simulink model "brain"  (Simulink 7.5)
settings: Solver=FixedStepDiscrete  StartTime=0.0  StopTime=inf  FixedStep=0.2  RelTol=1e-3
values from neighbouring files (symbols this model uses):
  Buoy1_Hue = 0.4    [brainconstants.m]    (also in brainconstants_David.m = 30)
  Buoy1_Saturation = 1.0    (= 1)    [brainconstants.m]    (also in brainconstants_David.m)
  Buoy1_Value = 0.45    [brainconstants.m]    (also in brainconstants_David.m)
  Buoy2_Hue = 0.0    (= 0)    [brainconstants.m]    (also in brainconstants_David.m = 80)
  Buoy2_Saturation = 1.0    (= 1)    [brainconstants.m]    (also in brainconstants_David.m)
  Buoy2_Value = 0.75    [brainconstants.m]    (also in brainconstants_David.m)
  Buoy_Max_Eccentricity = 0.7    [brainconstants.m]    (also in brainconstants_David.m = 1.2)
  Buoy_Max_Extent = 0.9    [brainconstants.m]    (also in brainconstants_David.m)
  Buoy_Min_Eccentricity = 0    [brainconstants.m]    (also in brainconstants_David.m)
  Buoy_Min_Extent = 0.7    [brainconstants.m]    (also in brainconstants_David.m = 0.1)
  Buoy_Strafe = 40    [brainconstants.m]    (also in brainconstants_David.m)
  Cam_Down_Strafe_XPos_Kd = 0.0    (= 0)    [brainconstants.m]    (also in brainconstants_David.m)
  Cam_Down_Strafe_XPos_Ki = 0.0    (= 0)    [brainconstants.m]    (also in brainconstants_David.m)
  Cam_Down_Strafe_XPos_Kp = -1.0    (= -1)    [brainconstants.m]    (also in brainconstants_David.m)
  Cam_Down_Yaw_XPos_Kd = 0.0    (= 0)    [brainconstants.m]    (also in brainconstants_David.m)
  Cam_Down_Yaw_XPos_Ki = 0.0    (= 0)    [brainconstants.m]    (also in brainconstants_David.m)
  Cam_Down_Yaw_XPos_Kp = 0.6    [brainconstants.m]    (also in brainconstants_David.m)
  Cam_Down_YPos_Kd = 0.0    (= 0)    [brainconstants.m]    (also in brainconstants_David.m)
  Cam_Down_YPos_Ki = 0.0    (= 0)    [brainconstants.m]    (also in brainconstants_David.m)
  Cam_Down_YPos_Kp = 0.75    [brainconstants.m]    (also in brainconstants_David.m)
  Cam_Forward_XPosition_Kd = 0.0    (= 0)    [brainconstants.m]    (also in brainconstants_David.m)
  Cam_Forward_XPosition_Ki = 0.0    (= 0)    [brainconstants.m]    (also in brainconstants_David.m)
  Cam_Forward_XPosition_Kp = 0.07    [brainconstants.m]    (also in brainconstants_David.m)
  Cam_Forward_YPosition_Kd = 0.0    (= 0)    [brainconstants.m]    (also in brainconstants_David.m)
  Cam_Forward_YPosition_Ki = 0.0    (= 0)    [brainconstants.m]    (also in brainconstants_David.m)
  Cam_Forward_YPosition_Kp = 0.8    [brainconstants.m]    (also in brainconstants_David.m)
  Depth_Kd = 0.0    (= 0)    [brainconstants.m]    (also in brainconstants_David.m)
  Depth_Ki = 0.0    (= 0)    [brainconstants.m]    (also in brainconstants_David.m)
  Depth_Kp = 75    [brainconstants.m]    (also in brainconstants_David.m)
  Heading_Forward_Velocity = 30    [brainconstants.m]    (also in brainconstants_David.m)
  Heading_Kd = 0.4    [brainconstants.m]    (also in brainconstants_David.m)
  Heading_Ki = 0.0    (= 0)    [brainconstants.m]    (also in brainconstants_David.m)
  Heading_Kp = 0.65    [brainconstants.m]    (also in brainconstants_David.m)
  Hedge_Hue = .4    (= 0.4)    [brainconstants.m]    (also in brainconstants_David.m)
  Hedge_Saturation = 1    [brainconstants.m]    (also in brainconstants_David.m)
  Hedge_Value = .75    (= 0.75)    [brainconstants.m]    (also in brainconstants_David.m)
  Iter_Segment_Thresh = 60    [brainconstants.m]    (also in brainconstants_David.m)
  MissionPlan = [1 1 1 1 1 1 1 1 1 1 1 1 1 0 0 0 0 0 0 0]    [brainconstants.m]    (also in brainconstants_David.m)
  Track_Desired_Depth = 8    [brainconstants.m]    (also in brainconstants_David.m)
  Track_HueHigher = 0.75    [brainconstants.m]    (also in brainconstants_David.m)
  Track_HueLower = 0.4    [brainconstants.m]    (also in brainconstants_David.m)
  Track_Min_Eccentricity = 0.9    [brainconstants.m]    (also in brainconstants_David.m)
  Track_Saturation = 0.75    [brainconstants.m]    (also in brainconstants_David.m)
  Vision_Forward_Velocity = 15    [brainconstants.m]    (also in brainconstants_David.m)
undefined symbols (not defined in the file or in its folder): DiscIntNeverNeededParam, gray, Rec, SDTV, strel, YawRate_Kd, YawRate_Ki, YawRate_Kp
libraries: vipconversions x32, simulink x26, vipgeotforms x9, vipstatistics x9, viptextngfix x7, vipmorphops x6, viptransforms x4, vipsnks x3, vipsrcs x1
(part 5 of 6)

== matlab function Normalize Thrusters to 1 ==
  data: Tin input double; Tout output double
function Tout = NormalizeThrusters(Tin)
% This function changes the thrusters from int8's to doubles and puts them
% on a scale from -1 to 1

Tout = double(Tin)./128;

return

== matlab function StateFlow Functions/StateFlowFunctions.Buoys.FindBuoys.LookforBuoys/Blob Extraction ==
  data: LabelMatrix input double; Eccent output double; num_colors input double; Extent output double; TotalNum output double; Centroid output double
function [Eccent,Extent,TotalNum,Centroid] = GetBlobInfo(LabelMatrix, num_colors)
% This function will determine the characteristics of the blobs in an image
% given a label matrix defining the different binary images contained in a
% that label matrix

[rows, cols] = size(LabelMatrix);
LogicMatrix = false(rows,cols);

max_num_blobs = 50;
min_blob_area = 5;

Centroid = zeros(max_num_blobs,2);
Eccent = zeros(1,max_num_blobs);
Extent = zeros(1,max_num_blobs);

TotalNum = uint8(0);

persistent hblob
if isempty(hblob)
    hblob = video.BlobAnalysis('AreaOutputPort',false,'BoundingBoxOutputPort',false,...
        'CentroidOutputPort',true,'EccentricityOutputPort',true,'ExtentOutputPort',true,...
        'NumBlobsOutputPort',true,'MinimumBlobAreaSource','Property',...
        'MinimumBlobArea', min_blob_area);
end

for k = 1:num_colors
    for i = 1:rows
        for j = 1:cols
            if(LabelMatrix(i,j) ~= k)
                LogicMatrix(i,j) = false;
            else
                LogicMatrix(i,j) = true;
            end
        end
    end
    [TCentroid,TEccent,TExtent,TNumBlobs] = step(hblob,LogicMatrix);
    
    if(TotalNum+TNumBlobs < max_num_blobs)
        for i = 1:TNumBlobs
            Centroid(TotalNum+i,1) = TCentroid(1,i);
            Centroid(TotalNum+i,2) = TCentroid(2,i);
            Eccent(TotalNum+i) = TEccent(i);
            Extent(TotalNum+i) = TExtent(i);
        end
        TotalNum = TotalNum + TNumBlobs;
    end
end

return

== matlab function StateFlow Functions/StateFlowFunctions.Buoys.FindBuoys.LookforBuoys/IF Buoy Conditions ==
  data: Eccent input double; Image output double; Extent input double; num_blobs input double; cent input double; Min_Eccent input double; Max_Eccent input double; Min_Extent input double; Max_Extent input double; BuoyCent output double
function [Image,BuoyCent] = BuoyConditions(Eccent,Extent,num_blobs, cent,Min_Eccent, Max_Eccent,Min_Extent,Max_Extent)
% This function will take in 2 1x10 vectors, eccent and extent to determine
% if there is a buoy present in the current image

Image = 0;
count = 0;
BuoyCent = ones(2,50);

for i = 1:num_blobs
    if((Eccent(i)>Min_Eccent) && (Eccent(i)<Max_Eccent) && (Extent(i)>Min_Extent) && (Extent(i)<Max_Extent))
        count = count + 1;
        BuoyCent(1,count) = cent(i,1);
        BuoyCent(2,count) = cent(i,2);
    end
end

if(count >= 3)
    Image = 1;
end

return

== matlab function StateFlow Functions/StateFlowFunctions.Buoys.FindBuoys.GetBuoyColors/Blob Extraction ==
  data: LabelMatrix input double; Eccent output double; num_colors input double; Extent output double; Centroid output double; TotalNum output double; Area output double
function [Eccent,Extent,Centroid,TotalNum,Area] = GetBlobInfo(LabelMatrix, num_colors)
% This function will determine the characteristics of the blobs in an image
% given a label matrix defining the different binary images contained in a
% that label matrix

[rows, cols] = size(LabelMatrix);
LogicMatrix = false(rows,cols);

max_num_blobs = 50;
min_blob_area = 10;

Area = zeros(1,max_num_blobs);
Centroid = zeros(max_num_blobs,2);
Eccent = zeros(1,max_num_blobs);
Extent = zeros(1,max_num_blobs);

TotalNum = uint8(0);

persistent hblob
if isempty(hblob)
    hblob = video.BlobAnalysis('AreaOutputPort',true,'BoundingBoxOutputPort',false,...
        'CentroidOutputPort',true,'EccentricityOutputPort',true,'ExtentOutputPort',true,...
        'NumBlobsOutputPort',true,'MinimumBlobAreaSource','Property',...
        'MinimumBlobArea', min_blob_area);
end

for k = 1:num_colors
    for i = 1:rows
        for j = 1:cols
            if(LabelMatrix(i,j) ~= k)
                LogicMatrix(i,j) = false;
            else
                LogicMatrix(i,j) = true;
            end
        end
    end
    [TArea, TCentroid,TEccent,TExtent,TNumBlobs] = step(hblob,LogicMatrix);
    
    if(TNumBlobs+TotalNum < max_num_blobs)
        for i = 1:TNumBlobs
            Area(TotalNum+i) = TArea(i);
            Centroid(TotalNum+i,1) = TCentroid(1,i);
            Centroid(TotalNum+i,2) = TCentroid(2,i);
            Eccent(TotalNum+i) = TEccent(i);
            Extent(TotalNum+i) = TExtent(i);
        end
        TotalNum = TotalNum + TNumBlobs;
    end
end

return

== matlab function StateFlow Functions/StateFlowFunctions.FollowOnePath.OnePath.AlignWithPath.GetHeadings/GetHeadingToPath ==
  data: Theta input double; Rho input double; Votes input double; AlongPathHeading output double
function AlongPathHeading   = GetHeading(Theta, Rho, Votes)
% This function calculates the heading to the path from Theta and Rho

numlines = floor(length(Theta)/2);

AlongPathHeading = -999*ones(1,numlines);
maxIndex = -999*ones(1,numlines);
most_votes = -999*ones(1,numlines);

[most_votes(1) maxIndex(1)] = max(Votes);
Votes(maxIndex(1)) = 0;
count = 1;

while(count < numlines)
    count = count + 1;
    [most_votes(count) maxIndex(count)] = max(Votes);
    Votes(maxIndex(count)) = 0;
end

for k = 1:numlines
    if(Theta(maxIndex(k)) > -90*pi()/180 && Theta(maxIndex(k)) < 90*pi()/180)
        AlongPathHeading(k) = Theta(maxIndex(k))*180/pi();
    end
end

cow = 1;

return

== matlab function StateFlow Functions/StateFlowFunctions.Buoys.FindBuoys.GetBuoyColors/IF Buoy Conditions ==
  data: Eccent input double; Centroid_Out output double; Extent input double; num_blobs input double; Min_Eccent input double; Max_Eccent input double; Min_Extent input double; Max_Extent input double; Centroids input double; count output double
function [Centroid_Out, count] = BuoyConditions(Eccent,Extent,num_blobs,Min_Eccent, Max_Eccent,Min_Extent,Max_Extent,Centroids)
% This function will take in 2 1x10 vectors, eccent and extent to determine
% the cenroids of the most circular objects in the image

count = 0;
Centroid_Out = zeros(50,2);


for i = 1:num_blobs
    if((Eccent(i)>Min_Eccent) && (Eccent(i)<Max_Eccent) && (Extent(i)>Min_Extent) && (Extent(i)<Max_Extent))
        count = count + 1;
        Centroid_Out(count,1) = Centroids(i,1);
        Centroid_Out(count,2) = Centroids(i,2);
    end
end

return

== matlab function StateFlow Functions/StateFlowFunctions.Buoys.FindBuoys.GetBuoyColors/Say Which Buoy Is Which ==
  data: LabelMatrix input double; blobs output double; ref_colors input double; Centroids input double; Areas input double; num_blobs input double
function blobs  = WhichBuoyIsWhich(LabelMatrix,ref_colors,Centroids,Areas, num_blobs)
% This function determines which buoy is in which location, left, middle,
% or right.

max_num_blobs = 50;
colors = zeros(max_num_blobs,3);
centX = zeros(1,max_num_blobs);
centY = zeros(1,max_num_blobs);
reference = zeros(1,1);
blobs = zeros(max_num_blobs,4);

for i = 1:num_blobs
    centX(i) = floor(Centroids(i,2));
    centY(i) = floor(Centroids(i,1));
    if(centX(i) < 1)
        centX(i) = 1;
    end
    if(centY(i) < 1)
        centY(i) = 1;
    end
    
    reference = LabelMatrix(centY(i),centX(i));
    
    colors(i,1:3) = [ref_colors(reference,1), ref_colors(reference,2), ref_colors(reference,3)];
end

% Putting blobs in order from left to right
for i = 1:num_blobs
    [value ref] = min(centX);
    blobs(i,1) = colors(ref,1);
    blobs(i,2) = colors(ref,2);
    blobs(i,3) = colors(ref,3);
    blobs(i,4) = Areas(ref);
    centX(ref) = 1000;
end

return

== matlab function StateFlow Functions/StateFlowFunctions.FollowOnePath.OnePath.CenterOver_Strafe/Embedded MATLAB Function ==
  data: Area1 input double; Centroid1 input double; BlobCentroidX output double; BlobCentroidY output double; Image input double
function [BlobCentroidX, BlobCentroidY] = PickBiggestBlob(Area1, Centroid1, Image)
% This function will choose and return data about the largest/left blob 
% given a set of blobs

if(Centroid1(1,1) == -1 && Centroid1(2,1) == -1)
    [ImageY ImageX] = size(Image);
    BlobCentroidX = floor(ImageX/2);
    BlobCentroidY = floor(ImageY/2);
    BlobArea = -1;
else
    [BlobArea, index] = max(double(Area1));
    Area1(index) = 0;
    [BlobArea2, index2] = max(double(Area1));
    
    if(BlobArea < BlobArea2*1.25)
        if(Centroid1(2,index) > Centroid1(2,index2))
            BlobCentroidX = Centroid1(2,index2);
            BlobCentroidY = Centroid1(1,index2);
        else
            BlobCentroidX = Centroid1(2,index);
            BlobCentroidY = Centroid1(1,index);
        end
    else
        BlobCentroidX = Centroid1(2,index);
        BlobCentroidY = Centroid1(1,index);
    end
end

return

== matlab function StateFlow Functions/StateFlowFunctions.FollowOnePath.OnePath.CenterOver_Strafe/Embedded MATLAB Function1 ==
  data: Image input double; XCenter output double; YCenter output double
function [XCenter,YCenter] = GetImageCenter(Image)
% This function finds the center of an image

[rows cols] = size(Image);

XCenter = floor(cols/2);
YCenter = floor(rows/2);

return

== matlab function StateFlow Functions/StateFlowFunctions.FollowOnePath.RecognizePath.LookforTrack/LookforTrack/CheckConditions ==
  data: Eccent input double; Image output double; Track_Min_Eccentricity input double
function Image = CheckConditions(Eccent, Track_Min_Eccentricity)
% This function checks the conditions to decide if a track is present

if(Eccent > Track_Min_Eccentricity)
    Image = 1;
else
    Image = 0;
end

return

== matlab function StateFlow Functions/StateFlowFunctions.FollowOnePath.MakeHSVImage/PutHSVImageTogether ==
  data: H input double; HSVImage1 output double; S input double; V input double
function HSVImage1 = PutHSVImageTogether(H,S,V)
% This function simply makes an HSV image a single multidimensional
% signal

[rows, cols] = size(H);

HSVImage1 = zeros(rows,cols,3);

HSVImage1(:,:,1) = H;
HSVImage1(:,:,2) = S;
HSVImage1(:,:,3) = V;

return

== matlab function StateFlow Functions/StateFlowFunctions.JumpHedge.ApproachHedge.GetArea/Embedded MATLAB Function ==
  data: Area1 input double; BlobArea output double; Image input double
function BlobArea  = PickBiggestBlob(Area1, Image)
% This function will choose and return data about the largest blob given a 
% set of blobs

if(Area1(1) == -1)
    [ImageY ImageX] = size(Image);
    BlobArea = -1;
else
    [BlobArea, index] = max(double(Area1));
end

return

== matlab function StateFlow Functions/StateFlowFunctions.Buoys.IterativeSegmentation/Low Pass Filter/Low Pass Filter ==
  data: I input double; Iout output double
function Iout = GaussianBlurr(I)
% This function calculates the gaussian blur of an intensity image

sigma = sqrt(2);

Grows = 3;    % Gaussian matrix rows
Gcols = 3;    % Gaussian matrix columns

[Irows Icols] = size(I);

Iout = single(zeros(Irows,Icols));

Trows = Irows - Grows + 1;
Tcols = Icols - Gcols + 1;
Itemp = single(zeros(Trows,Tcols));

G = zeros(Grows,Gcols);

FirstRow = ceil(-Grows/2);
LastRow = floor(Grows/2);
FirstCol = ceil(-Gcols/2);
LastCol = floor(Gcols/2);
Gsum = 0;
for i=FirstRow:LastRow
    for j = FirstCol:LastCol
        G(i-FirstRow+1,j-FirstCol+1) = exp(-(j*j+i*i)/(2*sigma*sigma));
        Gsum = Gsum + G(i-FirstRow+1,j-FirstCol+1);
    end
end

G = G./Gsum;

Itemp = conv2(single(I),single(G),'valid');

% reflect boundaries to keep image the same size
% top
Iout((1:LastRow),(LastCol+1:Icols-LastCol)) = Itemp((1:LastRow),(1:Tcols));
% bottom
Iout((Irows-LastRow+1:Irows),(LastCol+1:Icols-LastCol)) = Itemp((Trows-LastRow+1:Trows),(1:Tcols));
% left
Iout((1+LastRow:Irows-LastRow),(1:LastCol)) = Itemp((1:Trows),(1:LastCol));
% right
Iout((1+LastRow:Irows-LastRow),(Icols-LastCol+1:Icols)) = Itemp((1:Trows),(Tcols-LastCol+1:Tcols));
% center
Iout((1+LastRow:Irows-LastRow),(1+LastCol:Icols-LastCol)) = Itemp;
% top left corner
Iout(1:LastRow,1:LastCol) = Itemp(1:LastRow,1:LastCol);
% top right corner
Iout(1:LastRow,Icols-LastCol:Icols) = Itemp(1:LastRow,Tcols-LastCol:Tcols);
% bottom left corner
Iout(Irows-LastRow:Irows,1:LastCol) = Itemp(Trows-LastRow:Trows,1:LastCol);
% bottom right corner
Iout(Irows-LastRow:Irows,Icols-LastCol:Icols) = Itemp(Trows-LastRow:Trows,Tcols-LastCol:Tcols);

return

== matlab function StateFlow Functions/StateFlowFunctions.Buoys.ApproachBuoys.FindSecondBuoy.SecondBuoy/IF Buoy Conditions ==
  data: Cent input double; Eccent input double; Image output double; Extent input double; num_blobs input double; Min_Eccent input double; Max_Eccent input double; Min_Extent input double; Max_Extent input double; BlobPos output double
function [Image,BlobPos] = BuoyConditions(Cent,Eccent,Extent,num_blobs,Min_Eccent, Max_Eccent,Min_Extent,Max_Extent)
% This function will take in 2 1x10 vectors, eccent and extent to determine
% if there is a buoy present in the current image

Image = 0;
count = 0;
BlobPos = ones(2,1);

for i = 1:num_blobs
    if((Eccent(i)>Min_Eccent) && (Eccent(i)<Max_Eccent) && (Extent(i)>Min_Extent) && (Extent(i)<Max_Extent))
        Image = 1;
        BlobPos(1) = Cent(1,i);
        BlobPos(2) = Cent(2,i);
    end
end

return

== matlab function StateFlow Functions/StateFlowFunctions.Buoys.ApproachBuoys.FindSecondBuoy.SecondBuoy/Threshold The Image/Choose Closest Color ==
  data: ref_colors input double; index output double; num_colors input double; L input double; a input double; b input double
function index = GetColorIndex(ref_colors,num_colors,L,a,b)
% This function chooses the appropriate color option from the reference colors
% and set of desired L,a,b values

threshold = 70;

min_dist = 1000;
index = int8(num_colors+1);


for i = 1:num_colors
    dist = sqrt(2*(L-ref_colors(i,1))^2 + (a-ref_colors(i,2))^2 + (b-ref_colors(i,3))^2);
    if(dist < min_dist && dist < threshold)         % L: 0 - 100,a: -100 - 100 , b: -100 - 100
        min_dist = dist;                            % max min_dist = 346 if L dist is doubled
        index = int8(i);                            % max min_dist = 300 if L dist is not doubled
    end
end

return

== matlab function StateFlow Functions/StateFlowFunctions.Buoys.IterativeSegmentation/Low Pass Filter/Low Pass Filter1 ==
  data: I input double; Iout output double
function Iout = GaussianBlurr(I)
% This function calculates the gaussian blur of an intensity image

sigma = sqrt(2);

Grows = 3;    % Gaussian matrix rows
Gcols = 3;    % Gaussian matrix columns

[Irows Icols] = size(I);

Iout = single(zeros(Irows,Icols));

Trows = Irows - Grows + 1;
Tcols = Icols - Gcols + 1;
Itemp = single(zeros(Trows,Tcols));

G = zeros(Grows,Gcols);

FirstRow = ceil(-Grows/2);
LastRow = floor(Grows/2);
FirstCol = ceil(-Gcols/2);
LastCol = floor(Gcols/2);
Gsum = 0;
for i=FirstRow:LastRow
    for j = FirstCol:LastCol
        G(i-FirstRow+1,j-FirstCol+1) = exp(-(j*j+i*i)/(2*sigma*sigma));
        Gsum = Gsum + G(i-FirstRow+1,j-FirstCol+1);
    end
end

G = G./Gsum;

Itemp = conv2(single(I),single(G),'valid');

% reflect boundaries to keep image the same size
% top
Iout((1:LastRow),(LastCol+1:Icols-LastCol)) = Itemp((1:LastRow),(1:Tcols));
% bottom
Iout((Irows-LastRow+1:Irows),(LastCol+1:Icols-LastCol)) = Itemp((Trows-LastRow+1:Trows),(1:Tcols));
% left
Iout((1+LastRow:Irows-LastRow),(1:LastCol)) = Itemp((1:Trows),(1:LastCol));
% right
Iout((1+LastRow:Irows-LastRow),(Icols-LastCol+1:Icols)) = Itemp((1:Trows),(Tcols-LastCol+1:Tcols));
% center
Iout((1+LastRow:Irows-LastRow),(1+LastCol:Icols-LastCol)) = Itemp;
% top left corner
Iout(1:LastRow,1:LastCol) = Itemp(1:LastRow,1:LastCol);
% top right corner
Iout(1:LastRow,Icols-LastCol:Icols) = Itemp(1:LastRow,Tcols-LastCol:Tcols);
% bottom left corner
Iout(Irows-LastRow:Irows,1:LastCol) = Itemp(Trows-LastRow:Trows,1:LastCol);
% bottom right corner
Iout(Irows-LastRow:Irows,Icols-LastCol:Icols) = Itemp(Trows-LastRow:Trows,Tcols-LastCol:Tcols);

return

== matlab function StateFlow Functions/StateFlowFunctions.ValidationGate.LookforTrack/LookforTrack/CheckConditions ==
  data: Eccent input double; Image output double; Track_Min_Eccentricity input double
function Image = CheckConditions(Eccent, Track_Min_Eccentricity)
% This function checks the conditions to decide if a track is present

if(Eccent > Track_Min_Eccentricity)
    Image = 1;
else
    Image = 0;
end

return

== matlab function StateFlow Functions/StateFlowFunctions.Buoys.ApproachBuoys.ApproachFirstBuoy.WhichBuoysToApproach/GetBestColorMatch ==
  data: Buoys input double; B1_L input double; B1_a input double; B1_b input double; B2_L input double; B2_a input double; B2_b input double; Direction1 output double; num_blobs input double; Direction2 output double
function [Direction1, Direction2] = GetBestColorMatch(Buoys,B1_L,B1_a,B1_b,B2_L,B2_a,B2_b,num_blobs)
% This function determines which buoys are the best match for the desired colors

% Buoys = zeros(3,3);
% Buoys = [L;M;R];
min_dist = 1000;
min_dist2 = 1000;
FirstD = 2+zeros(1,50);
SecondD = 2+zeros(1,50);

count1 = 0;
count2 = 0;

for i = 1:num_blobs
    dist = sqrt((Buoys(i,1) - B1_L)^2 + (Buoys(i,2) - B1_a)^2 + (Buoys(i,3) - B1_b)^2);
    if(dist <= min_dist)
        count1 = count1 + 1;
        min_dist = dist;
        FirstD(count1) = i;
    end
    dist2 = sqrt((Buoys(i,1) - B2_L)^2 + (Buoys(i,2) - B2_a)^2 + (Buoys(i,3) - B2_b)^2);
    if(dist2 < min_dist2)
        count2 = count2 + 1;
        min_dist2 = dist2;
        SecondD(count2) = i;
    end
end

Index1 = 2;
largest_buoyarea1 = 0;
for i = 1:count1
    buoyarea = Buoys(FirstD(i),4);
    if(buoyarea > largest_buoyarea1)
        Index1 = FirstD(i);
        largest_buoyarea = buoyarea;
    end
end

Index2 = 2;
largest_buoyarea2 = 0;
for i = 1:count2
    buoyarea = Buoys(SecondD(i),4);
    if(buoyarea > largest_buoyarea2)
        Index2 = SecondD(i);
        largest_buoyarea = buoyarea;
    end
end

if(Index1 > Index2)
    Direction1 = 1;
    Direction2 = 3;
elseif(Index1 == Index2)
    Direction1 = 2;
    Direction2 = 2;
else
    Direction1 = 3;
    Direction2 = 1;
end

return

== matlab function StateFlow Functions/StateFlowFunctions.Buoys.ApproachBuoys.Buoy/Embedded MATLAB Function ==
  data: Area1 input double; Centroid1 input double; Eccent1 input double; MinE input double; BlobArea output double; BlobCentroidX output double; BlobCentroidY output double; Image input double
function [BlobArea, BlobCentroidX, BlobCentroidY] = PickBestBlob(Area1,Centroid1,Eccent1,MinE, Image)
% This function will choose and return data about the blob most similar to
% the desired set of characteristics given a set of blobs

DesiredE = MinE;

% Determine closest blob to desired Eccentricity
Dist = abs(Eccent1 - MinE);

if(Centroid1(1,1) == -1 && Centroid1(2,1) == -1)
    [ImageY ImageX] = size(Image);
    BlobCentroidX = floor(ImageX/2);
    BlobCentroidY = floor(ImageY/2);
    BlobArea = -1;
else
    [MinDist, index] = min(double(Dist));
    Dist(index) = 2;
    [MinDist2,index2] = min(double(Dist));
    
    if(MinDist2 < MinDist * 1.5)
        if(Centroid1(2,index) >= Centroid1(2,index2))
            BlobCentroidX = Centroid1(2, index);
            BlobCentroidY = Centroid1(1, index);
            BlobArea = double(Area1(index));
        else
            BlobCentroidX = Centroid1(2, index2);
            BlobCentroidY = Centroid1(1, index2);
            BlobArea = double(Area1(index2));
        end
    else
        BlobCentroidX = Centroid1(2, index);
        BlobCentroidY = Centroid1(1, index);
        BlobArea = double(Area1(index));
    end
end

return

== matlab function StateFlow Functions/StateFlowFunctions.Buoys.IterativeSegmentation/Low Pass Filter/Low Pass Filter2 ==
  data: I input double; Iout output double
function Iout = GaussianBlurr(I)
% This function calculates the gaussian blur of an intensity image

sigma = sqrt(2);

Grows = 3;    % Gaussian matrix rows
Gcols = 3;    % Gaussian matrix columns

[Irows Icols] = size(I);

Iout = single(zeros(Irows,Icols));

Trows = Irows - Grows + 1;
Tcols = Icols - Gcols + 1;
Itemp = single(zeros(Trows,Tcols));

G = zeros(Grows,Gcols);

FirstRow = ceil(-Grows/2);
LastRow = floor(Grows/2);
FirstCol = ceil(-Gcols/2);
LastCol = floor(Gcols/2);
Gsum = 0;
for i=FirstRow:LastRow
    for j = FirstCol:LastCol
        G(i-FirstRow+1,j-FirstCol+1) = exp(-(j*j+i*i)/(2*sigma*sigma));
        Gsum = Gsum + G(i-FirstRow+1,j-FirstCol+1);
    end
end

G = G./Gsum;

Itemp = conv2(single(I),single(G),'valid');

% reflect boundaries to keep image the same size
% top
Iout((1:LastRow),(LastCol+1:Icols-LastCol)) = Itemp((1:LastRow),(1:Tcols));
% bottom
Iout((Irows-LastRow+1:Irows),(LastCol+1:Icols-LastCol)) = Itemp((Trows-LastRow+1:Trows),(1:Tcols));
% left
Iout((1+LastRow:Irows-LastRow),(1:LastCol)) = Itemp((1:Trows),(1:LastCol));
% right
Iout((1+LastRow:Irows-LastRow),(Icols-LastCol+1:Icols)) = Itemp((1:Trows),(Tcols-LastCol+1:Tcols));
% center
Iout((1+LastRow:Irows-LastRow),(1+LastCol:Icols-LastCol)) = Itemp;
% top left corner
Iout(1:LastRow,1:LastCol) = Itemp(1:LastRow,1:LastCol);
% top right corner
Iout(1:LastRow,Icols-LastCol:Icols) = Itemp(1:LastRow,Tcols-LastCol:Tcols);
% bottom left corner
Iout(Irows-LastRow:Irows,1:LastCol) = Itemp(Trows-LastRow:Trows,1:LastCol);
% bottom right corner
Iout(Irows-LastRow:Irows,Icols-LastCol:Icols) = Itemp(Trows-LastRow:Trows,Tcols-LastCol:Tcols);

return

== matlab function StateFlow Functions/StateFlowFunctions.JumpHedge.RecognizeHedge.LookForHedge/Are 3 Lines Present ==
  data: HoughTable input double; Image output double; T output double; Theta input double; Rho input double; R output double
function [Image,T,R] = AreLinesPresent(HoughTable,Theta,Rho)
% This function is meant to see if there are 3 lines which approximate a
% 'hedge' in the current frame

R = zeros(1,3);
T = zeros(1,3);
[rhos, thetas] = size(HoughTable);

% Find the two vetical lines
theta_0_col = floor(thetas/2);

most_votes = 0;
second_most = 0;
indexi1 = 1;
indexi2 = 1;
indexj1 = 1;
indexj2 = 1;

for i = 1:rhos
    for j = theta_0_col-5:theta_0_col+5
        if(HoughTable(i,j) > most_votes)
            if(abs(Rho(indexi1)-Rho(i)) > 20)
                second_most = HoughTable(indexi1,indexj2);
                indexi2 = indexi1;
                indexj2 = indexj1;
                R(2) = R(1);
                T(2) = T(1);
            end
            most_votes = HoughTable(i,j);
            indexi1 = i;
            indexj1 = j;
            R(1) = Rho(i);
            T(1) = Theta(j);
        elseif(HoughTable(i,j) > second_most && abs(Rho(indexi1)-Rho(i)) > 20)
            second_most = HoughTable(i,j);
            indexi2 = i;
            indexj2 = j;
            R(2) = Rho(i);
            T(2) = Theta(j);
        end
    end
end

% Find the horizontal line
max_votes = 0;
index = [0 0];
for i = 1:rhos
    for j = 1:10
        if(HoughTable(i,j) > max_votes)
            max_votes = HoughTable(i,j);
            index = [i,j];
            R(3) = Rho(i);
            T(3) = Theta(j);
        end
    end
    for j = thetas-10:thetas
        if(HoughTable(i,j) > max_votes)
            max_votes = HoughTable(i,j);
            index = [i,j];
            R(3) = Rho(i);
            T(3) = Theta(j);
        end
    end
end

% Find the most prominent line
top_vote = 0;
t = 0;
r = 0;
for i = 1:rhos
    for j = 1:thetas
        if(HoughTable(i,j) > top_vote)
            top_vote = HoughTable(i,j);
            t = j;
            r = i;
        end
    end
end

Image = 0;
if(top_vote*.75 < max_votes && top_vote*.3 < most_votes && top_vote*.3 < second_most)
    Image = 1;
end

cow = 1;

return

== matlab function StateFlow Functions/StateFlowFunctions.Buoys.ApproachBuoys.Buoy/Embedded MATLAB Function1 ==
  data: Image input double; XCenter output double; YCenter output double
function [XCenter,YCenter] = GetImageCenter(Image)
% This function finds the center of an image

[rows cols] = size(Image);

XCenter = floor(cols/2);
YCenter = floor(rows/2);

return

== matlab function StateFlow Functions/StateFlowFunctions.Buoys.ApproachBuoys.Buoy/Threshold The Image/Choose Closest Color ==
  data: ref_colors input double; index output double; num_colors input double; L input double; a input double; b input double
function index = GetColorIndex(ref_colors,num_colors,L,a,b)
% This function chooses the appropriate color option from the reference colors
% and set of desired L,a,b values

min_dist = 1000;

x = 1;
y = 1.5;
z = 1.5;

index = int8(1);
for i = 1:num_colors
    dist = sqrt(x*(L-ref_colors(i,1))^2 + y*(a-ref_colors(i,2))^2 + z*(b-ref_colors(i,3))^2);
    if(dist < min_dist)
        min_dist = dist;
        index = int8(i);
    end
end

return

== matlab function StateFlow Functions/StateFlowFunctions.Buoys.ShowSegmentedImage/Embedded MATLAB Function ==
  data: LabMatrix input double; L output double; Ref_Colors input double; a output double; b output double
function [L,a,b]=CombineSegmentedImage(LabMatrix,Ref_Colors)
% This function puts together the segmented imaged such that it can be shown

[rows, cols] = size(LabMatrix);
L = zeros(rows,cols);
a = zeros(rows,cols);
b = zeros(rows,cols);

for i = 1:rows
    for j = 1:cols
        L(i,j) = Ref_Colors(LabMatrix(i,j),1);
        a(i,j) = Ref_Colors(LabMatrix(i,j),2);
        b(i,j) = Ref_Colors(LabMatrix(i,j),3);
    end
end

return

== matlab function StateFlow Functions/StateFlowFunctions.Buoys.ShowSegmentedImage/Embedded MATLAB Function1 ==
  data: R input double; RGB output double; G input double; B input double
function RGB = SeparatetoSingleSignals(R,G,B)
% This function combines the separate color signals into a single 3-D signal

[rows, cols] = size(R);

RGB = zeros(rows,cols,3);

for i = 1:rows
    for j = 1:cols
        RGB(i,j,1) = R(i,j);
        RGB(i,j,2) = G(i,j);
        RGB(i,j,3) = B(i,j);
    end
end

return

== matlab function StateFlow Functions/StateFlowFunctions.Buoys.IterativeSegmentation/Segmentation/LabSegmentation ==
  data: L input double; LabelMatrix output double; a input double; b input double; ref_colors input double; num_colors input double
function LabelMatrix  = LabSegmentation(L,a,b,ref_colors,num_colors)
% This function generates the label matrix

[rows cols] = size(L);

Lout = zeros(rows,cols);
aout = zeros(rows,cols);
bout = zeros(rows,cols);

LabelMatrix = zeros(rows,cols);

for i = 1:rows
    for j = 1:cols
        min_dist = 1000;
        index = 1;
        for k = 1:num_colors
            dist = sqrt((ref_colors(k,1) - L(i,j))^2 + (ref_colors(k,2) - a(i,j))^2 + (ref_colors(k,3) - b(i,j))^2);
            if(dist < min_dist)
                min_dist = double(dist);
                index = k;
            end
        end
        LabelMatrix(i,j) = index;
    end
end

for i = 1:rows
    for j = 1:cols
        Lout(i,j) = ref_colors(LabelMatrix(i,j),1);
        aout(i,j) = ref_colors(LabelMatrix(i,j),2);
        bout(i,j) = ref_colors(LabelMatrix(i,j),3);
    end
end

cow = 1;

return

== matlab function StateFlow Functions/StateFlowFunctions.Buoys.IterativeSegmentation/Segmentation/Reference Color Selection ==
  data: L input double; ref_colors output double; a input double; b input double; num_colors output double; Dist_Thresh input double
function [ref_colors, num_colors] = Segmentation(L,a,b,Dist_Thresh)
% This function tries segmentation by adding new reference colors everytime
% a pixel is found with a distance greater than a certain amount from
% every other reference color

[rows cols] = size(L);

Dist_Threshold = Dist_Thresh;% L = 0 to 100, a = -100 to 100, b = -100 to 100
                    % max dist = 300 -> 60/300 is 20%
x = 1;  % coefficients determining distance calculation
y = 1.5;
z = 1.5;

max_num_colors = 50;
ref_colors = zeros(max_num_colors,3);   % At most 50 different reference colors
LabelMatrix = zeros(rows,cols);
num_colors = 1;

center_row = floor(rows/2);
center_col = floor(cols/2);

ref_colors(1,:) = [L(center_row,center_col) a(center_row,center_col) b(center_row,center_col)];

flag = 0;
i = 1;
j = 1;
while(i <= rows)        % perform initial segmentation
    while(i <= rows && flag == 0)
        while(j <= cols && flag == 0)
            k = 1;
            min_dist = 1000;
            index = 1;
            while(k <= num_colors)
                dist = sqrt(x*(ref_colors(k,1) - L(i,j))^2 + y*(ref_colors(k,2) - a(i,j))^2 + z*(ref_colors(k,3) - b(i,j))^2);
                if(min_dist > dist)
                    min_dist = double(dist);
                    index = k;
                end
                k = k + 1;
            end
            if(j == 117)
                cow = 1;
            end
            if(min_dist > Dist_Threshold && num_colors < max_num_colors)
                ref_colors(num_colors+1,:) = [L(i,j) a(i,j) b(i,j)];
                num_colors = num_colors + 1;
                flag = 1;
                i = 0;
                j = 0;
            else
                LabelMatrix(i,j) = index;
            end
            j = j + 1;
        end
        j = 1;
        i = i + 1;
    end
    flag = 0;
end

% Go through image once more to get more accurate values for the different regions
ref_color_L_avg = zeros(50,1);
ref_color_a_avg = zeros(50,1);
ref_color_b_avg = zeros(50,1);
color_count = zeros(50,1);
for i = 1:rows
    for j = 1:cols
        index = LabelMatrix(i,j);
        ref_color_L_avg(index) = ref_color_L_avg(index) + L(i,j);
        ref_color_a_avg(index) = ref_color_a_avg(index) + a(i,j);
        ref_color_b_avg(index) = ref_color_b_avg(index) + b(i,j);
        color_count(index) = color_count(index) + 1;
    end
end
ref_color_L_avg = ref_color_L_avg ./ color_count;
ref_color_a_avg = ref_color_a_avg ./ color_count;
ref_color_b_avg = ref_color_b_avg ./ color_count;

for i = 1:num_colors
    ref_colors(i,1) = ref_color_L_avg(i);
    ref_colors(i,2) = ref_color_a_avg(i);
    ref_colors(i,3) = ref_color_b_avg(i);
end

return

== matlab function StateFlow Functions/StateFlowFunctions.FollowOnePath.OnePath.AlignWithPath.Align/Embedded MATLAB Function ==
  data: HeadingAlong input double; PIDoutput input double; Strafe output double
function Strafe = CheckHeadingAlong(HeadingAlong,PIDoutput)
% This function makes sure the path was seen and if not, the only sends the
% forward command to the thrusters

if(HeadingAlong == -999)
    Strafe = 0;
else
    Strafe = PIDoutput;
end

return

== matlab function StateFlow Functions/StateFlowFunctions.FollowOnePath.OnePath.AlignWithPath.GetHeadings/Hough Transform Stuff/IsLinePresent ==
  data: HoughTable input double; Theta output double; ThetaValues input double; RhoValues input double; Rho output double; maxVotes output double
function [Theta,Rho, maxVotes]  = IsLinePresent(HoughTable, ThetaValues, RhoValues)
% This function takes a Hough/hash table as input and  determines if a line
% is present and if so what its Rho and Theta are.

num_lines = 2;

minVotes = 15;

Rho = -999*ones(1,num_lines);
Theta = -999*ones(1,num_lines);
maxVotes = -999*ones(1,num_lines);
ThetaIndex = -999*ones(1,num_lines);
RhoIndex = -999*ones(1,num_lines);

[num_rho num_theta] = size(HoughTable);

index = 1;

[maxValues RhoIndices] = max(HoughTable);
[maxVotes(index) ThetaIndex(index)] = max(maxValues);
index_moment = 0;
sum_maxValues = 0;
for i = 1:num_theta
    if(maxVotes(index) - maxValues(i) < 0.15*maxVotes(index))
        index_moment = i*maxValues(i) + index_moment;
        sum_maxValues = sum_maxValues + maxValues(i);
    end
end
if(sum_maxValues > 0)
    best_index = round(index_moment/sum_maxValues); 
else
    best_index = 1;
end

ThetaIndex(index) = best_index;
maxVotes(index) = maxValues(best_index);

RhoIndex(index) = RhoIndices(ThetaIndex(index));

if(maxVotes(1) >= minVotes)
    HoughTable(RhoIndex(index),ThetaIndex(index)) = 0;
    if(num_lines > 1)
        index = index + 1;
        count = 0;
        while(index <= num_lines && count < num_lines+10)
            count = count + 1;
            [maxValues RhoIndices] = max(HoughTable);
            [maxVotes(index) ThetaIndex(index)] = max(maxValues);
            RhoIndex(index) = RhoIndices(ThetaIndex(index));
            
            HoughTable(RhoIndex(index),ThetaIndex(index)) = 0;
            
            if(abs(RhoIndex(index)-RhoIndex(index-1))>20 || abs(ThetaIndex(index)-ThetaIndex(index-1))>30)
                index = index + 1;
            end
        end
    end
    
    for index = 1:num_lines
        if(maxVotes(index) > minVotes)
            Theta(index) = ThetaValues(ThetaIndex(index));
            Rho(index) = RhoValues(RhoIndex(index));
            if(Theta(index) > 0 && Rho(index) < 0)
                Rho(index) = Rho(index) * -1;
            end
        end
    end
end

cow = 1;

return

== matlab function StateFlow Functions/StateFlowFunctions.JumpHedge.ShowSegmentedImage/Embedded MATLAB Function ==
  data: LabMatrix input double; L output double; Ref_Colors input double; a output double; b output double
function [L,a,b]=CombineSegmentedImage(LabMatrix,Ref_Colors)
% This function puts together the segmented imaged such that it can be shown

[rows, cols] = size(LabMatrix);
L = zeros(rows,cols);
a = zeros(rows,cols);
b = zeros(rows,cols);

for i = 1:rows
    for j = 1:cols
        L(i,j) = Ref_Colors(LabMatrix(i,j),1);
        a(i,j) = Ref_Colors(LabMatrix(i,j),2);
        b(i,j) = Ref_Colors(LabMatrix(i,j),3);
    end
end

return

== matlab function StateFlow Functions/StateFlowFunctions.JumpHedge.ShowSegmentedImage/Embedded MATLAB Function1 ==
  data: R input double; RGB output double; G input double; B input double
function RGB = SeparatetoSingleSignals(R,G,B)
% This function combines the separate color signals into a single 3-D signal

[rows, cols] = size(R);

RGB = zeros(rows,cols,3);

for i = 1:rows
    for j = 1:cols
        RGB(i,j,1) = R(i,j);
        RGB(i,j,2) = G(i,j);
        RGB(i,j,3) = B(i,j);
    end
end

return

== matlab function StateFlow Functions/StateFlowFunctions.JumpHedge.CameraForward_CenterOnBlobYaw/Embedded MATLAB Function ==
  data: Area1 input double; BlobArea output double; Centroid1 input double; BlobCentroidX output double; BlobCentroidY output double; Image input double
function [BlobArea, BlobCentroidX, BlobCentroidY] = PickBiggestBlob(Area1, Centroid1, Image)
% This function will choose and return data about the largest blob given a 
% set of blobs

if(Centroid1(1,1) == -1 && Centroid1(2,1) == -1)
    [ImageY ImageX] = size(Image);
    BlobCentroidX = floor(ImageX/2);
    BlobCentroidY = floor(ImageY/2);
    BlobArea = -1;
else
    [BlobArea, index] = max(double(Area1));
    BlobCentroidX = Centroid1(2, index);
    BlobCentroidY = Centroid1(1, index);
end

return

== matlab function StateFlow Functions/StateFlowFunctions.JumpHedge.CameraForward_CenterOnBlobYaw/Embedded MATLAB Function1 ==
  data: Image input double; XCenter output double; YCenter output double
function [XCenter,YCenter] = GetImageCenter(Image)
% This function finds the center of an image

[rows cols] = size(Image);

XCenter = floor(cols/2);
YCenter = floor(rows/2);

return

== matlab function StateFlow Functions/StateFlowFunctions.JumpHedge.GetAxisRatio/Embedded MATLAB Function ==
  data: Area1 input double; BlobArea output double; BBox input double; AxisRatio output double; Image input double
function [BlobArea, AxisRatio] = PickBiggestBlob(Area1, BBox, Image)
% This function will choose and return data about the largest blob given a 
% set of blobs

if(BBox(1,1) == -1)
    [ImageY ImageX] = size(Image);
    AxisRatio = 0;
    BlobArea = -1;
else
    [BlobArea, index] = max(double(Area1));
    AxisRatio = double(BBox(4,index))/double(BBox(3,index));
end

return

== matlab function StateFlow Functions/StateFlowFunctions.JumpHedge.IndividualSegmentation/Threshold The Image/Choose Closest Color ==
  data: ref_colors input double; index output double; num_colors input double; L input double; a input double; b input double
function index = GetColorIndex(ref_colors,num_colors,L,a,b)
% This function chooses the appropriate color option from the reference colors
% and set of desired L,a,b values

min_dist = 1000;
max_dist = 100;

x = 1;
y = 1.5;
z = 1.5;

index = int8(1);
for i = 1:num_colors
    dist = sqrt(x*(L-ref_colors(i,1))^2 + y*(a-ref_colors(i,2))^2 + z*(b-ref_colors(i,3))^2);
    if(dist < min_dist)
        min_dist = dist;
        index = int8(i);
    end
end

if(min_dist > max_dist)
    index = int8(num_colors+1);
end

return

== matlab function StateFlow Functions/StateFlowFunctions.JumpHedge.IterativeSegmentation/Low Pass Filter/Low Pass Filter ==
  data: I input double; Iout output double
function Iout = GaussianBlurr(I)
% This function calculates the gaussian blur of an intensity image

sigma = sqrt(2);

Grows = 3;    % Gaussian matrix rows
Gcols = 3;    % Gaussian matrix columns

[Irows Icols] = size(I);

Iout = single(zeros(Irows,Icols));

Trows = Irows - Grows + 1;
Tcols = Icols - Gcols + 1;
Itemp = single(zeros(Trows,Tcols));

G = zeros(Grows,Gcols);

FirstRow = ceil(-Grows/2);
LastRow = floor(Grows/2);
FirstCol = ceil(-Gcols/2);
LastCol = floor(Gcols/2);
Gsum = 0;
for i=FirstRow:LastRow
    for j = FirstCol:LastCol
        G(i-FirstRow+1,j-FirstCol+1) = exp(-(j*j+i*i)/(2*sigma*sigma));
        Gsum = Gsum + G(i-FirstRow+1,j-FirstCol+1);
    end
end

G = G./Gsum;

Itemp = conv2(single(I),single(G),'valid');

% reflect boundaries to keep image the same size
% top
Iout((1:LastRow),(LastCol+1:Icols-LastCol)) = Itemp((1:LastRow),(1:Tcols));
% bottom
Iout((Irows-LastRow+1:Irows),(LastCol+1:Icols-LastCol)) = Itemp((Trows-LastRow+1:Trows),(1:Tcols));
% left
Iout((1+LastRow:Irows-LastRow),(1:LastCol)) = Itemp((1:Trows),(1:LastCol));
% right
Iout((1+LastRow:Irows-LastRow),(Icols-LastCol+1:Icols)) = Itemp((1:Trows),(Tcols-LastCol+1:Tcols));
% center
Iout((1+LastRow:Irows-LastRow),(1+LastCol:Icols-LastCol)) = Itemp;
% top left corner
Iout(1:LastRow,1:LastCol) = Itemp(1:LastRow,1:LastCol);
% top right corner
Iout(1:LastRow,Icols-LastCol:Icols) = Itemp(1:LastRow,Tcols-LastCol:Tcols);
% bottom left corner
Iout(Irows-LastRow:Irows,1:LastCol) = Itemp(Trows-LastRow:Trows,1:LastCol);
% bottom right corner
Iout(Irows-LastRow:Irows,Icols-LastCol:Icols) = Itemp(Trows-LastRow:Trows,Tcols-LastCol:Tcols);

return

== matlab function StateFlow Functions/StateFlowFunctions.JumpHedge.IterativeSegmentation/Low Pass Filter/Low Pass Filter1 ==
  data: I input double; Iout output double
function Iout = GaussianBlurr(I)
% This function calculates the gaussian blur of an intensity image

sigma = sqrt(2);

Grows = 3;    % Gaussian matrix rows
Gcols = 3;    % Gaussian matrix columns

[Irows Icols] = size(I);

Iout = single(zeros(Irows,Icols));

Trows = Irows - Grows + 1;
Tcols = Icols - Gcols + 1;
Itemp = single(zeros(Trows,Tcols));

G = zeros(Grows,Gcols);

FirstRow = ceil(-Grows/2);
LastRow = floor(Grows/2);
FirstCol = ceil(-Gcols/2);
LastCol = floor(Gcols/2);
Gsum = 0;
for i=FirstRow:LastRow
    for j = FirstCol:LastCol
        G(i-FirstRow+1,j-FirstCol+1) = exp(-(j*j+i*i)/(2*sigma*sigma));
        Gsum = Gsum + G(i-FirstRow+1,j-FirstCol+1);
    end
end

G = G./Gsum;

Itemp = conv2(single(I),single(G),'valid');

% reflect boundaries to keep image the same size
% top
Iout((1:LastRow),(LastCol+1:Icols-LastCol)) = Itemp((1:LastRow),(1:Tcols));
% bottom
Iout((Irows-LastRow+1:Irows),(LastCol+1:Icols-LastCol)) = Itemp((Trows-LastRow+1:Trows),(1:Tcols));
% left
Iout((1+LastRow:Irows-LastRow),(1:LastCol)) = Itemp((1:Trows),(1:LastCol));
% right
Iout((1+LastRow:Irows-LastRow),(Icols-LastCol+1:Icols)) = Itemp((1:Trows),(Tcols-LastCol+1:Tcols));
% center
Iout((1+LastRow:Irows-LastRow),(1+LastCol:Icols-LastCol)) = Itemp;
% top left corner
Iout(1:LastRow,1:LastCol) = Itemp(1:LastRow,1:LastCol);
% top right corner
Iout(1:LastRow,Icols-LastCol:Icols) = Itemp(1:LastRow,Tcols-LastCol:Tcols);
% bottom left corner
Iout(Irows-LastRow:Irows,1:LastCol) = Itemp(Trows-LastRow:Trows,1:LastCol);
% bottom right corner
Iout(Irows-LastRow:Irows,Icols-LastCol:Icols) = Itemp(Trows-LastRow:Trows,Tcols-LastCol:Tcols);

return

== matlab function StateFlow Functions/StateFlowFunctions.JumpHedge.IterativeSegmentation/Low Pass Filter/Low Pass Filter2 ==
  data: I input double; Iout output double
function Iout = GaussianBlurr(I)
% This function calculates the gaussian blur of an intensity image

sigma = sqrt(2);

Grows = 3;    % Gaussian matrix rows
Gcols = 3;    % Gaussian matrix columns

[Irows Icols] = size(I);

Iout = single(zeros(Irows,Icols));

Trows = Irows - Grows + 1;
Tcols = Icols - Gcols + 1;
Itemp = single(zeros(Trows,Tcols));

G = zeros(Grows,Gcols);

FirstRow = ceil(-Grows/2);
LastRow = floor(Grows/2);
FirstCol = ceil(-Gcols/2);
LastCol = floor(Gcols/2);
Gsum = 0;
for i=FirstRow:LastRow
    for j = FirstCol:LastCol
        G(i-FirstRow+1,j-FirstCol+1) = exp(-(j*j+i*i)/(2*sigma*sigma));
        Gsum = Gsum + G(i-FirstRow+1,j-FirstCol+1);
    end
end

G = G./Gsum;

Itemp = conv2(single(I),single(G),'valid');

% reflect boundaries to keep image the same size
% top
Iout((1:LastRow),(LastCol+1:Icols-LastCol)) = Itemp((1:LastRow),(1:Tcols));
% bottom
Iout((Irows-LastRow+1:Irows),(LastCol+1:Icols-LastCol)) = Itemp((Trows-LastRow+1:Trows),(1:Tcols));
% left
Iout((1+LastRow:Irows-LastRow),(1:LastCol)) = Itemp((1:Trows),(1:LastCol));
% right
Iout((1+LastRow:Irows-LastRow),(Icols-LastCol+1:Icols)) = Itemp((1:Trows),(Tcols-LastCol+1:Tcols));
% center
Iout((1+LastRow:Irows-LastRow),(1+LastCol:Icols-LastCol)) = Itemp;
% top left corner
Iout(1:LastRow,1:LastCol) = Itemp(1:LastRow,1:LastCol);
% top right corner
Iout(1:LastRow,Icols-LastCol:Icols) = Itemp(1:LastRow,Tcols-LastCol:Tcols);
% bottom left corner
Iout(Irows-LastRow:Irows,1:LastCol) = Itemp(Trows-LastRow:Trows,1:LastCol);
% bottom right corner
Iout(Irows-LastRow:Irows,Icols-LastCol:Icols) = Itemp(Trows-LastRow:Trows,Tcols-LastCol:Tcols);

return

== matlab function StateFlow Functions/StateFlowFunctions.JumpHedge.IterativeSegmentation/Segmentation/LabSegmentation ==
  data: L input double; LabelMatrix output double; a input double; b input double; ref_colors input double; num_colors input double
function LabelMatrix  = LabSegmentation(L,a,b,ref_colors,num_colors)
% This function generates the label matrix

[rows cols] = size(L);

Lout = zeros(rows,cols);
aout = zeros(rows,cols);
bout = zeros(rows,cols);

LabelMatrix = zeros(rows,cols);

for i = 1:rows
    for j = 1:cols
        min_dist = 1000;
        index = 1;
        for k = 1:num_colors
            dist = sqrt((ref_colors(k,1) - L(i,j))^2 + (ref_colors(k,2) - a(i,j))^2 + (ref_colors(k,3) - b(i,j))^2);
            if(dist < min_dist)
                min_dist = double(dist);
                index = k;
            end
        end
        LabelMatrix(i,j) = index;
    end
end

for i = 1:rows
    for j = 1:cols
        Lout(i,j) = ref_colors(LabelMatrix(i,j),1);
        aout(i,j) = ref_colors(LabelMatrix(i,j),2);
        bout(i,j) = ref_colors(LabelMatrix(i,j),3);
    end
end

cow = 1;

return
